simulink model "pendulum1"  (R2023a)
settings: Solver=FixedStepAuto  StartTime=0.0  StopTime=10.0  FixedStep=0.001  RelTol=1e-3
values from neighbouring files (symbols this model uses):
  g = 9.81    [pendulum.m]
  L = length_pendulam_values(i)    [pendulum.m]
  thetadot = 45    [pendulum.m]
settings Model: Creator=alaam  LastModifiedBy=alaam

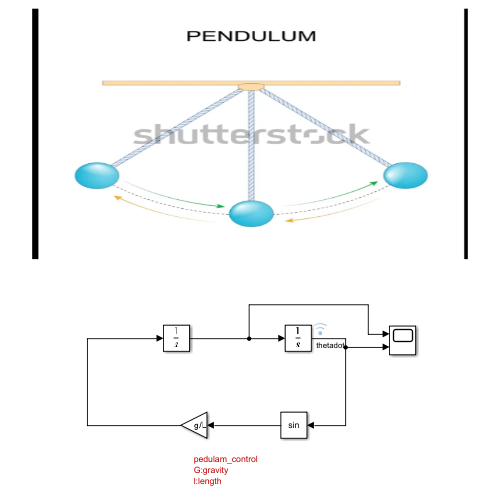
[thumbnail: Simulink's stored preview of the top-level diagram]
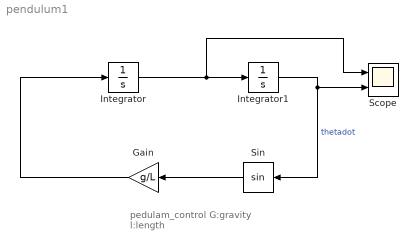
== system pendulum1 ==
  note: pedulam_control
      | G:gravity
      | l:length
  Gain : Gain  Gain=g/L
  Integrator : Integrator
  Integrator1 : Integrator  InitialCondition=thetadot
  Scope : Scope  NumInputPorts=2
  Sin : Trigonometry
  wires:
  Integrator/1 -> Scope/1, Integrator1/1
  Gain/1 -> Integrator/1
  Integrator1/1 -> Sin/1, Scope/2  "thetadot"
  Sin/1 -> Gain/1
